simulink model "pitch_angle_design_step"  (R2019b)
settings: Solver=FixedStepAuto  StartTime=0.0  StopTime=step_sim_time  RelTol=1e-3
values from neighbouring files (symbols this model uses):
  disturb = 1    [rootlocus.m]
  disturb_time = 20    [rootlocus.m]
  Kp_pa = 3    [rootlocus.m]
  step_time = 0    [rootlocus.m]
settings Model: Creator=francois  LastModifiedBy=francois

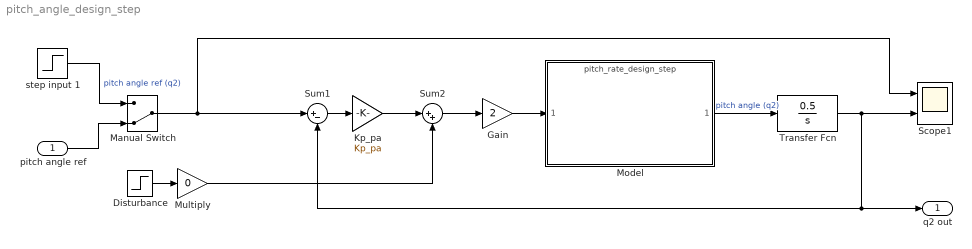
== system pitch_angle_design_step ==
  "pitch angle ref " : Inport
  "Disturbance " : Step  Time=disturb_time  After=disturb  SampleTime=0
  Gain : Gain  Gain=2
  "Kp_pa " : Gain  Gain=Kp_pa
  Manual Switch : ManualSwitch  CurrentSetting=0
  Model : ModelReference  ModelNameDialog=pitch_rate_design_step.slx  SimulationMode=Normal  ModelReferenceVersion=1.17
  Multiply : Gain  Gain=0
  Scope1 : Scope  NumInputPorts=2
  Sum1 : Sum  Inputs=|+-
  Sum2 : Sum  Inputs=|++
  Transfer Fcn : TransferFcn  Numerator=[0.5]  Denominator=[1 0]
  step input 1 : Step  Time=step_time  SampleTime=0
  "q2 out " : Outport  SignalName=q2 out
  wires:
  Sum1/1 -> "Kp_pa "/1
  Transfer Fcn/1 -> "q2 out "/1, Sum1/2, Scope1/2
  Gain/1 -> Model/1
  "Kp_pa "/1 -> Sum2/1
  Sum2/1 -> Gain/1
  Model/1 -> Transfer Fcn/1  "pitch angle (q2)"
  "Disturbance "/1 -> Multiply/1
  Multiply/1 -> Sum2/2
  Manual Switch/1 -> Scope1/1, Sum1/1
  step input 1/1 -> Manual Switch/1  "pitch angle ref (q2)"
  "pitch angle ref "/1 -> Manual Switch/2
